simulink library "TestingLibrary_boy"  (R2018b)
settings: Solver=VariableStepAuto  StartTime=0.0  StopTime=10.0  RelTol=1e-3
undefined symbols (not defined in the file): B_eci_unit, e2sun_eci_unit, ECLIPSE, env_acc_mps2, sc2sun_eci_unit, simParams
libraries: $bdroot x2, gravityGrad_Lib x1, atmoDrag_lib x1, magField_lib x1, solarPressure_lib x1, clock_lib x1, orbit_data_bus x1, time_Lib x1
settings Model: Creator=Taylor  LastModifiedBy=devantormey

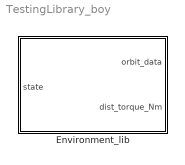
== system TestingLibrary_boy ==
  Environment_lib : Subsystem

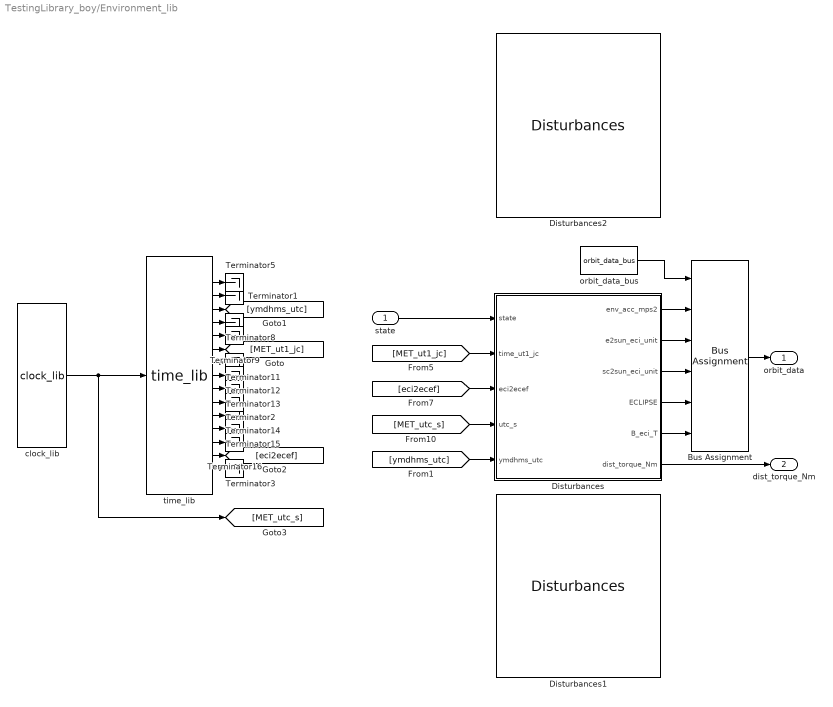
== system TestingLibrary_boy/Environment_lib ==
  state : Inport
  Bus Assignment : BusAssignment  AssignedSignals=env_acc_mps2,e2sun_eci_unit,sc2sun_eci_unit,ECLIPSE,B_eci_unit
  Disturbances : Subsystem
  Disturbances1 : $bdroot/Environment_lib/Disturbances  SystemSampleTime=-1
  Disturbances2 : $bdroot/Environment_lib/Disturbances  SystemSampleTime=-1
  Terminator{1..3,5,8..9,11..16} (12 alike) : Terminator
  clock_lib : clock_lib/clock_lib  SystemSampleTime=-1
  orbit_data_bus : orbit_data_bus/orbit_data_bus  SystemSampleTime=-1
  "time_lib " : time_Lib/time_lib    SystemSampleTime=-1
  orbit_data : Outport
  dist_torque_Nm : Outport  Port=2
  wires:
  [MET_utc_s] -> Disturbances/4(utc_s)
  Disturbances/5(B_eci_T) -> Bus Assignment/6
  Disturbances/2(e2sun_eci_unit) -> Bus Assignment/3
  "time_lib "/4 -> Terminator8/1
  [MET_ut1_jc] -> Disturbances/2(time_ut1_jc)
  Disturbances/3(sc2sun_eci_unit) -> Bus Assignment/4
  "time_lib "/3 -> [ymdhms_utc]
  [eci2ecef] -> Disturbances/3(eci2ecef)
  "time_lib "/5 -> Terminator9/1
  clock_lib/1 -> [MET_utc_s], "time_lib "/1
  Disturbances/6(dist_torque_Nm) -> dist_torque_Nm/1
  "time_lib "/1 -> Terminator5/1
  [ymdhms_utc] -> Disturbances/5(ymdhms_utc)
  Disturbances/4(ECLIPSE) -> Bus Assignment/5
  Disturbances/1(env_acc_mps2) -> Bus Assignment/2
  state/1 -> Disturbances/1(state)
  orbit_data_bus/1 -> Bus Assignment/1
  Bus Assignment/1 -> orbit_data/1
  "time_lib "/2 -> Terminator1/1
  "time_lib "/6 -> [MET_ut1_jc]
  "time_lib "/7 -> Terminator11/1
  "time_lib "/8 -> Terminator12/1
  "time_lib "/9 -> Terminator13/1
  "time_lib "/10 -> Terminator2/1
  "time_lib "/11 -> Terminator14/1
  "time_lib "/12 -> Terminator15/1
  "time_lib "/13 -> Terminator16/1
  "time_lib "/14 -> [eci2ecef]
  "time_lib "/15 -> Terminator3/1

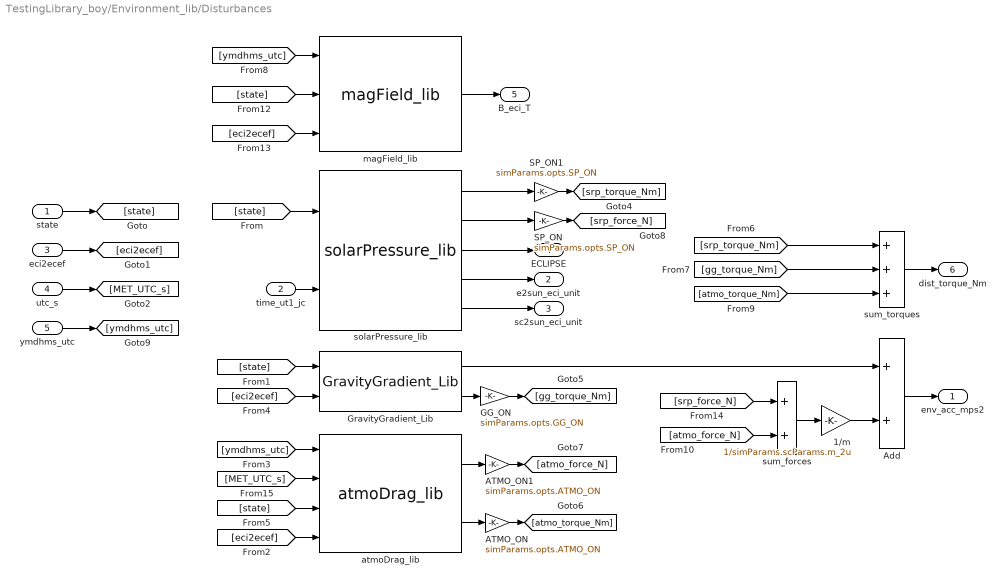
== system TestingLibrary_boy/Environment_lib/Disturbances ==
  state : Inport
  time_ut1_jc : Inport  Port=2
  eci2ecef : Inport  Port=3
  utc_s : Inport  Port=4
  ymdhms_utc : Inport  Port=5
  1/m : Gain  Gain=1/simParams.scParams.m_2u
  ATMO_ON : Gain  Gain=simParams.opts.ATMO_ON
  ATMO_ON1 : Gain  Gain=simParams.opts.ATMO_ON
  Add : Sum
  GG_ON : Gain  Gain=simParams.opts.GG_ON
  "GravityGradient_Lib " : gravityGrad_Lib/GravityGradient_Lib   SystemSampleTime=-1
  SP_ON : Gain  Gain=simParams.opts.SP_ON
  "SP_ON1 " : Gain  Gain=simParams.opts.SP_ON
  atmoDrag_lib : atmoDrag_lib/atmoDrag_lib  SystemSampleTime=-1
  magField_lib : magField_lib/magField_lib  SystemSampleTime=-1
      link override Rate Transition2: InitialCondition=0
  solarPressure_lib : solarPressure_lib/solarPressure_lib  SystemSampleTime=-1
  sum_forces : Sum
  sum_torques : Sum  Inputs=+++
  env_acc_mps2 : Outport
  e2sun_eci_unit : Outport  Port=2
  sc2sun_eci_unit : Outport  Port=3
  ECLIPSE : Outport  Port=4
  B_eci_T : Outport  Port=5
  dist_torque_Nm : Outport  Port=6
  wires:
  solarPressure_lib/3 -> ECLIPSE/1
  solarPressure_lib/1 -> "SP_ON1 "/1
  solarPressure_lib/4 -> e2sun_eci_unit/1
  solarPressure_lib/2 -> SP_ON/1
  time_ut1_jc/1 -> solarPressure_lib/2
  sum_forces/1 -> 1/m/1
  Add/1 -> env_acc_mps2/1
  1/m/1 -> Add/2
  atmoDrag_lib/2 -> ATMO_ON/1
  atmoDrag_lib/1 -> ATMO_ON1/1
  ATMO_ON/1 -> [atmo_torque_Nm]
  state/1 -> [state]
  [state] -> solarPressure_lib/1
  [state] -> "GravityGradient_Lib "/1
  eci2ecef/1 -> [eci2ecef]
  [eci2ecef] -> atmoDrag_lib/4
  [state] -> atmoDrag_lib/3
  utc_s/1 -> [MET_UTC_s]
  [ymdhms_utc] -> atmoDrag_lib/1
  [MET_UTC_s] -> atmoDrag_lib/2
  "SP_ON1 "/1 -> [srp_torque_Nm]
  [srp_torque_Nm] -> sum_torques/1
  GG_ON/1 -> [gg_torque_Nm]
  [gg_torque_Nm] -> sum_torques/2
  [eci2ecef] -> "GravityGradient_Lib "/2
  sum_torques/1 -> dist_torque_Nm/1
  [atmo_torque_Nm] -> sum_torques/3
  [atmo_force_N] -> sum_forces/2
  [srp_force_N] -> sum_forces/1
  ATMO_ON1/1 -> [atmo_force_N]
  SP_ON/1 -> [srp_force_N]
  "GravityGradient_Lib "/1 -> Add/1
  "GravityGradient_Lib "/2 -> GG_ON/1
  [state] -> magField_lib/2
  ymdhms_utc/1 -> [ymdhms_utc]
  [ymdhms_utc] -> magField_lib/1
  [eci2ecef] -> magField_lib/3
  magField_lib/1 -> B_eci_T/1
  solarPressure_lib/5 -> sc2sun_eci_unit/1
